simulink model "astolfi"  (R2021b)
settings: Solver=ode45  StartTime=0.0  StopTime=10  RelTol=1e-10
undefined symbols (not defined in the file or in its folder): KM, M11, M22
settings Model: Creator=mbober  LastModifiedBy=mbober

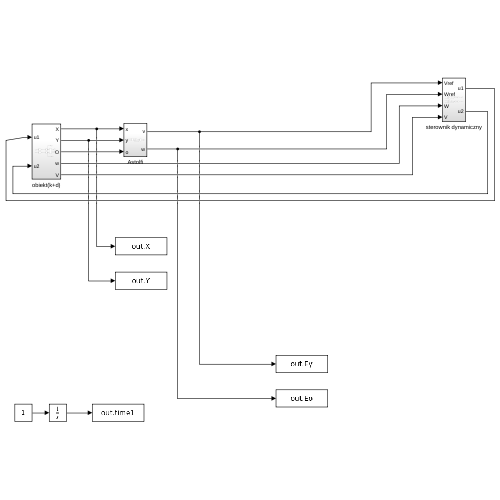
[thumbnail: Simulink's stored preview of the top-level diagram]
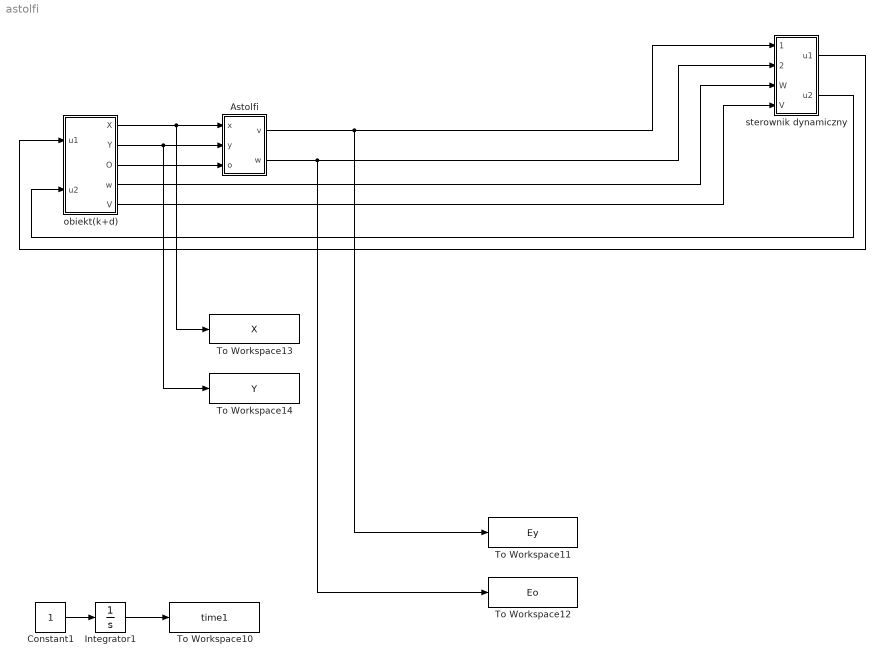
== system astolfi ==
  Astolfi : Subsystem
  Constant1 : Constant
  Integrator1 : Integrator
  To Workspace10 : ToWorkspace  VariableName=time1  SampleTime=-1
  To Workspace11 : ToWorkspace  VariableName=Ey  SampleTime=-1
  To Workspace12 : ToWorkspace  VariableName=Eo  SampleTime=-1
  To Workspace13 : ToWorkspace  VariableName=X  SampleTime=-1
  To Workspace14 : ToWorkspace  VariableName=Y  SampleTime=-1
  obiekt(k+d) : Subsystem
  sterownik dynamiczny : Subsystem
  wires:
  obiekt(k+d)/2(Y) -> Astolfi/2(y), To Workspace14/1
  sterownik dynamiczny/1(u1) -> obiekt(k+d)/1(u1)
  obiekt(k+d)/4(w) -> sterownik dynamiczny/3(W)
  Integrator1/1 -> To Workspace10/1
  obiekt(k+d)/5(V) -> sterownik dynamiczny/4(V)
  Astolfi/2(w) -> To Workspace12/1, sterownik dynamiczny/2(Wref)
  obiekt(k+d)/3(O) -> Astolfi/3(o)
  Astolfi/1(v) -> sterownik dynamiczny/1(Vref), To Workspace11/1
  obiekt(k+d)/1(X) -> Astolfi/1(x), To Workspace13/1
  sterownik dynamiczny/2(u2) -> obiekt(k+d)/2(u2)
  Constant1/1 -> Integrator1/1

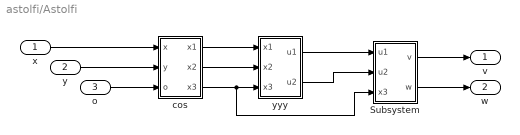
== system astolfi/Astolfi ==
  x : Inport
  y : Inport  Port=2
  o : Inport  Port=3
  Subsystem : Subsystem
  cos : Subsystem
  yyy : Subsystem
  v : Outport
  w : Outport  Port=2
  wires:
  cos/2(x2) -> yyy/2(x2)
  Subsystem/1(v) -> v/1
  x/1 -> cos/1(x)
  Subsystem/2(w) -> w/1
  y/1 -> cos/2(y)
  cos/1(x1) -> yyy/1(x1)
  o/1 -> cos/3(o)
  cos/3(x3) -> Subsystem/3(x3), yyy/3(x3)
  yyy/2(u2) -> Subsystem/2(u2)
  yyy/1(u1) -> Subsystem/1(u1)

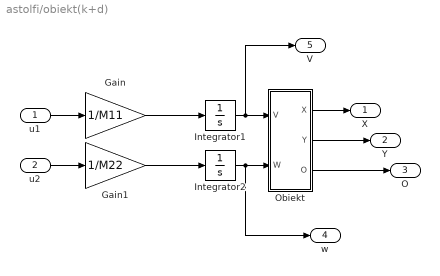
== system astolfi/obiekt(k+d) ==
  u1 : Inport
  u2 : Inport  Port=2
  Gain : Gain  Gain=1/M11
  Gain1 : Gain  Gain=1/M22
  Integrator1 : Integrator
  Integrator2 : Integrator
  Obiekt : Subsystem
  X : Outport
  Y : Outport  Port=2
  O : Outport  Port=3
  w : Outport  Port=4
  V : Outport  Port=5
  wires:
  Gain1/1 -> Integrator2/1
  Obiekt/1(X) -> X/1
  u1/1 -> Gain/1
  Integrator2/1 -> w/1, Obiekt/2(W)
  Integrator1/1 -> V/1, Obiekt/1(V)
  Gain/1 -> Integrator1/1
  Obiekt/2(Y) -> Y/1
  u2/1 -> Gain1/1
  Obiekt/3(O) -> O/1

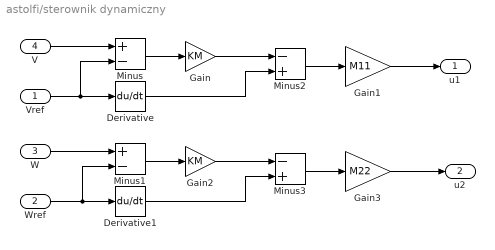
== system astolfi/sterownik dynamiczny ==
  Vref : Inport
  Wref : Inport  Port=2
  W : Inport  Port=3
  V : Inport  Port=4
  Derivative : Derivative
  Derivative1 : Derivative
  Gain : Gain  Gain=KM
  Gain1 : Gain  Gain=M11
  Gain2 : Gain  Gain=KM
  Gain3 : Gain  Gain=M22
  Minus : Sum  Inputs=+-
  Minus1 : Sum  Inputs=+-
  Minus2 : Sum  Inputs=-+
  Minus3 : Sum  Inputs=-+
  u1 : Outport
  u2 : Outport  Port=2
  wires:
  Minus3/1 -> Gain3/1
  Gain1/1 -> u1/1
  Minus1/1 -> Gain2/1
  Gain2/1 -> Minus3/1
  Minus2/1 -> Gain1/1
  Vref/1 -> Minus/2, Derivative/1
  Gain/1 -> Minus2/1
  Wref/1 -> Minus1/2, Derivative1/1
  Derivative1/1 -> Minus3/2
  V/1 -> Minus/1
  W/1 -> Minus1/1
  Derivative/1 -> Minus2/2
  Minus/1 -> Gain/1
  Gain3/1 -> u2/1

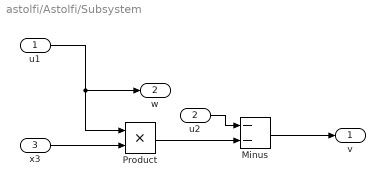
== system astolfi/Astolfi/Subsystem ==
  u1 : Inport
  u2 : Inport  Port=2
  x3 : Inport  Port=3
  Minus : Sum  Inputs=--
  Product : Product
  v : Outport
  w : Outport  Port=2
  wires:
  u2/1 -> Minus/1
  Product/1 -> Minus/2
  x3/1 -> Product/2
  u1/1 -> w/1, Product/1
  Minus/1 -> v/1

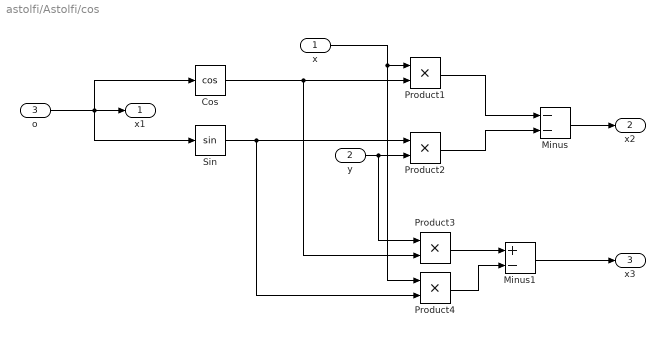
== system astolfi/Astolfi/cos ==
  x : Inport
  y : Inport  Port=2
  o : Inport  Port=3
  Cos : Trigonometry  Operator=cos
  Minus : Sum  Inputs=--
  Minus1 : Sum  Inputs=+-
  Product{1..4} (4 alike) : Product
  Sin : Trigonometry
  x1 : Outport
  x2 : Outport  Port=2
  x3 : Outport  Port=3
  wires:
  o/1 -> Sin/1, Cos/1, x1/1
  Minus/1 -> x2/1
  x/1 -> Product4/1, Product1/1
  Product1/1 -> Minus/1
  y/1 -> Product3/1, Product2/2
  Sin/1 -> Product4/2, Product2/1
  Product2/1 -> Minus/2
  Minus1/1 -> x3/1
  Product3/1 -> Minus1/1
  Product4/1 -> Minus1/2
  Cos/1 -> Product3/2, Product1/2

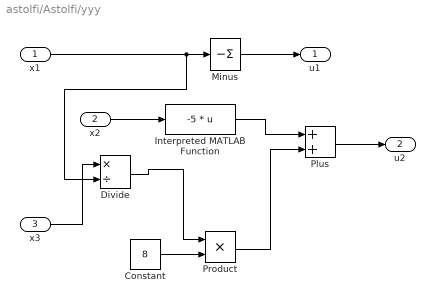
== system astolfi/Astolfi/yyy ==
  x1 : Inport
  x2 : Inport  Port=2
  x3 : Inport  Port=3
  Constant : Constant  Value=8
  Divide : Product  Inputs=*/
  Interpreted MATLAB Function : MATLABFcn  MATLABFcn=-5 * u
  Minus : Sum  Inputs=-
  Plus : Sum
  Product : Product
  u1 : Outport
  u2 : Outport  Port=2
  wires:
  x1/1 -> Divide/2, Minus/1
  Divide/1 -> Product/1
  Minus/1 -> u1/1
  x3/1 -> Divide/1
  x2/1 -> Interpreted MATLAB Function/1
  Plus/1 -> u2/1
  Interpreted MATLAB Function/1 -> Plus/1
  Constant/1 -> Product/2
  Product/1 -> Plus/2

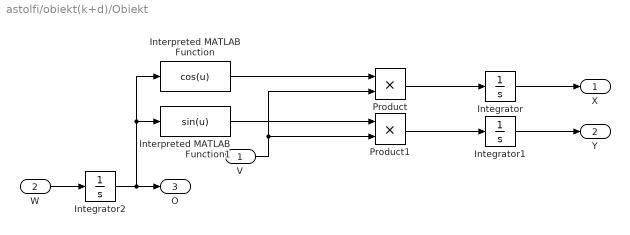
== system astolfi/obiekt(k+d)/Obiekt ==
  V : Inport
  W : Inport  Port=2
  Integrator : Integrator
  Integrator1 : Integrator
  Integrator2 : Integrator  InitialCondition=0.01
  Interpreted MATLAB Function : MATLABFcn  MATLABFcn=cos(u)
  Interpreted MATLAB Function1 : MATLABFcn  MATLABFcn=sin(u)
  Product : Product
  Product1 : Product
  X : Outport
  Y : Outport  Port=2
  O : Outport  Port=3
  wires:
  Product1/1 -> Integrator1/1
  Product/1 -> Integrator/1
  Integrator/1 -> X/1
  Integrator2/1 -> O/1, Interpreted MATLAB Function/1, Interpreted MATLAB Function1/1
  V/1 -> Product1/2, Product/2
  Integrator1/1 -> Y/1
  Interpreted MATLAB Function1/1 -> Product1/1
  W/1 -> Integrator2/1
  Interpreted MATLAB Function/1 -> Product/1
